simulink model "Original_example1_cs"  (R2018b)
settings: Solver=ode5  StartTime=0.0  StopTime=inf  FixedStep=1/20  RelTol=1e-3
PreLoadFcn:
  | mbxruntime.callbacks.PreLoadFcn(bdroot);
PostLoadFcn:
  | mbxruntime.callbacks.PostLoadFcn(bdroot);
InitFcn:
  | mbxruntime.callbacks.InitFcn(bdroot);
StartFcn:
  | mbxruntime.callbacks.StartFcn(bdroot);
StopFcn:
  | mbxruntime.callbacks.StopFcn(bdroot);
model workspace: external: MAT-File example1_cs_hws.mat (data not in the file)
undefined symbols (not defined in the file or in its folder): Broadcast, CameraTimestamp, Confidence, ConfidenceType, DiscIntNeverNeededParam, ErrorCode, Header, Height, Id, Id_SL_Info, InitImageOutputDir, Length, LidarTimestamp, PerceptionObstacle, PerceptionObstacle_SL_Info, PolygonPoint, PolygonPoint_SL_Info, Pose, Position, RadarTimestamp, S, SequenceNum, Theta, Timestamp, TimestampSec, TrackingTime, Type, Velocity, warningInitialVelocity, Waypoint, Waypoint_SL_Info, Width, X, x0, Y, Z
libraries: simulink x27, PreScanSimulinkLibrary x14, robotlib x12, simulink_extras x5, robotcorelib x2
(part 5 of 5)

== matlab function Original_example1_cs/BMW_X5_SUV_1/MATLAB Function ==
  data: Rotx input; RotationMatrix output; Roty input; Rotz input
function RotationMatrix = fcn(Rotx,Roty,Rotz)

Rx = [1,0,0; 0,cos(Rotx),-sin(Rotx); 0,sin(Rotx),cos(Rotx);];
Ry = [cos(Roty),0,sin(Roty); 0,1,0; -sin(Roty),0,cos(Roty);];
Rz = [cos(Rotz),-sin(Rotz),0; sin(Rotz),cos(Rotz),0; 0,0,1;];



RotationMatrix = Rx*Ry*Rz;

== matlab function Original_example1_cs/BMW_X5_SUV_1/PathFollower_Preview_1/LateralController/Calculate delta steering error/eml_delta_steering_error ==
  data: v_x_vehicle input; v_x_vehicle_Min input; t_Preview_LatCtrl input; delta_steeringwheeltotal output; v_y_vehicle input; yawrate_vehicle input; CorneringStiffness_Tyres_Front input; CorneringStiffness_Tyres_Rear input; m_vehicle_total input; inertia_z_vehicle_total input; e_Lat input size=10; Pos_x_CoG_Vehicle input; wheelbase input; RefreshCounter parameter
function delta_steeringwheeltotal = eml_delta_steering_error(v_x_vehicle,v_x_vehicle_Min,t_Preview_LatCtrl,v_y_vehicle,yawrate_vehicle,CorneringStiffness_Tyres_Front,CorneringStiffness_Tyres_Rear,m_vehicle_total,inertia_z_vehicle_total,e_Lat,Pos_x_CoG_Vehicle,wheelbase,RefreshCounter)

delta_steeringwheeltotal = emlfcn_delta_steering_error(v_x_vehicle,v_x_vehicle_Min,t_Preview_LatCtrl,v_y_vehicle,yawrate_vehicle,CorneringStiffness_Tyres_Front,CorneringStiffness_Tyres_Rear,m_vehicle_total,inertia_z_vehicle_total,e_Lat,Pos_x_CoG_Vehicle,wheelbase,RefreshCounter);

% end function

== matlab function Original_example1_cs/BMW_X5_SUV_1/MATLAB Function2 ==
  data: Euler input; Ex output; Ey output; Ez output
function [Ex,Ey,Ez]= fcn(Euler)

Ex = Euler(1,1);
Ey = Euler(2,1);
Ez = Euler(3,1);

== matlab function Original_example1_cs/BMW_X5_SUV_1/MATLAB Function1 ==
  data: Quat input; Qw output; Qx output; Qy output; Qz output
function [Qw,Qx,Qy,Qz]= fcn(Quat)

Qw = Quat(1,1);
Qx = Quat(2,1);
Qy = Quat(3,1);
Qz = Quat(4,1);
